simulink model "GSandFlareV2"  (R2021b)
settings: Solver=VariableStepAuto  StartTime=0.0  StopTime=10.0  RelTol=1e-3
values from neighbouring files (symbols this model uses):
  A_5 = SS_long_lo.A([1 2 3 4 5],[1 2 3 4 5])    [FindF16Dynamics.m]
  B_5 = SS_long_lo.A([1 2 3 4 5],[6 7])    [FindF16Dynamics.m]
  C_5 = SS_long_lo.C([1 2 3 4 5],[1 2 3 4 5])    [FindF16Dynamics.m]
  D_5 = SS_long_lo.D([1 2 3 4 5],[1 2])    [FindF16Dynamics.m]
  trim_alt = altitude    (= 5000)    [FindF16Dynamics.m]
  trim_thrust = trim_thrust_lo    [FindF16Dynamics.m]
  trim_velocity = velocity    (= 300)    [FindF16Dynamics.m]
undefined symbols (not defined in the file or in its folder): trim_state_lo
settings Model: Creator=Victor  LastModifiedBy=Victor

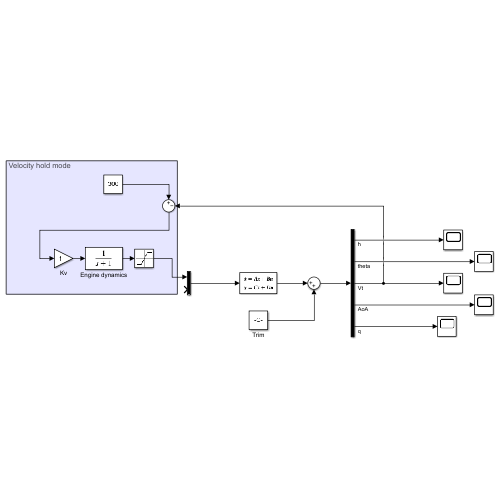
[thumbnail: Simulink's stored preview of the top-level diagram]
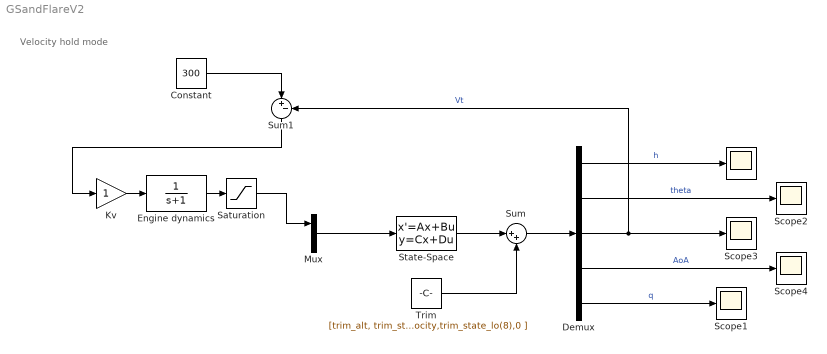
== system GSandFlareV2 ==
  note: Velocity hold mode
  " " : Scope
  Constant : Constant  Value=300
  Demux : Demux  Outputs=5
  Engine dynamics : TransferFcn  Denominator=[1 1]
  Kv : Gain
  Mux : Mux  Inputs=2
  Saturation : Saturate  UpperLimit=19000-trim_thrust  LowerLimit=1000-trim_thrust
  Scope{1..4} (4 alike) : Scope
  State-Space : StateSpace  A=A_5  B=B_5  C=C_5  D=D_5  InitialCondition=0
  Sum : Sum  Inputs=|++
  Sum1 : Sum  Inputs=|+-
  Trim : Constant  Value=[trim_alt, trim_state_lo(5), trim_velocity,trim_state_lo(8),0 ]
  wires:
  State-Space/1 -> Sum/1
  Demux/1 -> " "/1  "h"
  Demux/4 -> Scope4/1  "AoA"
  Demux/5 -> Scope1/1  "q"
  Trim/1 -> Sum/2
  Sum/1 -> Demux/1
  Demux/2 -> Scope2/1  "theta"
  Mux/1 -> State-Space/1
  Demux/3 -> Sum1/2, Scope3/1  "Vt"
  Constant/1 -> Sum1/1
  Kv/1 -> Engine dynamics/1
  Sum1/1 -> Kv/1
  Engine dynamics/1 -> Saturation/1
  Saturation/1 -> Mux/1
